simulink model "MDR_AA_TMD_Intercepteur"  (R2019b)
settings: Solver=ode4  StartTime=0.0  StopTime=Inf  FixedStep=0.01  RelTol=1e-3
values from neighbouring files (symbols this model uses):
  stdatm = [0 100 200 300 400 500 600 700 800 900 1000 1100 ... (4305 elements, 861x5)]    [stdatm.mat]
undefined symbols (not defined in the file or in its folder): Aero_Struct_CM, Aero_TMD, e0_0, e1_0, e2_0, e3_0, magnitude, Masse_Inertie_TMD, pow, Propu_TMD, Simu_TMD, Vm_0, xme_0
libraries: simulink x17
(part 1 of 4)
settings Model: Creator=julie  LastModifiedBy=julie

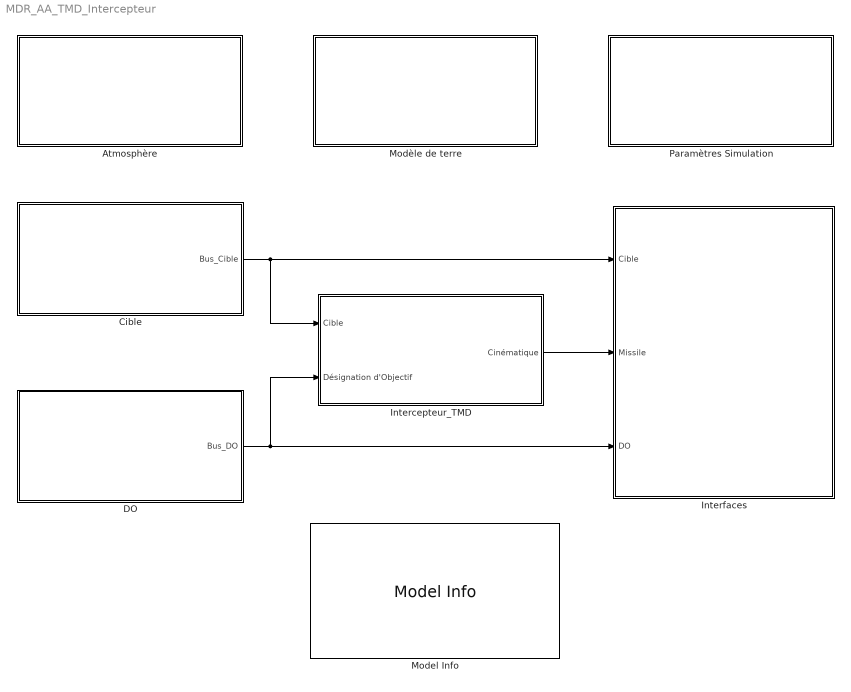
== system MDR_AA_TMD_Intercepteur ==
  Atmosphère : Subsystem
      mask Display: fprintf('Atmosphère')
  Cible : Subsystem  mask(Cible){}
      mask help: Evolution temporelle de la cible
      mask Display: fprintf('Cible')
  DO : Subsystem  mask(Cible){}
      mask help: Evolution temporelle de la DO
      mask Display: fprintf('Désignation d''Objectif')
  Intercepteur_TMD : Subsystem
      mask Display: fprintf('Missile')
  Interfaces : Subsystem
      mask Display: fprintf('Interfaces')
  Model Info : simulink/Model-Wide Utilities/Model Info  Frame=on  DisplayStringWithTags=|  HorizontalTextAlignment=Center  LeftAlignmentValue=0.5
      | Créé par Julien THADASACK
      | Modifié par 
      | %<ModifiedBy>
      | le 
      | %<ModifiedDate>
  Modèle de terre : Subsystem
      mask Display: fprintf('Modèle de terre')
  Paramètres Simulation : Subsystem
      mask Display: fprintf('Paramètres Simulation')
  wires:
  DO/1(Bus_DO) -> Intercepteur_TMD/2(Désignation d'Objectif), Interfaces/3(DO)
  Intercepteur_TMD/1(Cinématique) -> Interfaces/2(Missile)
  Cible/1(Bus_Cible) -> Intercepteur_TMD/1(Cible), Interfaces/1(Cible)

== system MDR_AA_TMD_Intercepteur/Atmosphère ==
  Atmosphère standard US76 : Subsystem  mask(Atmosphère standard US76){T_simu=-1}
      mask prompts: T_simu "Période de Simulation (s)"
      mask help: Recherche la pression, la température, la densité et la vitesse du son en fonction de l'altitude par rapport au niveau moyen de la mer.
      mask init:
      | load('stdatm');
      mask Help: eval('OpenHelp(''A3_NG.mdl'', ''\Help\html\A3_NG_Model_Atmosphere_US76.html'')');
  Bus Creator : BusCreator  Inputs=4
  Bus Selector : BusSelector  OutputSignals=Xi
  Selector : Selector  InputPortWidth=3  IndexOptions=Index vector (dialog)  Indices=[3]  OutputSizes=1
  Z positif vers le bas sinon : Gain  Gain=-1
  tag scope: Global_Atm=global
  wires:
  Atmosphère standard US76/3(Rho) -> Bus Creator/3  "Rho"
  Atmosphère standard US76/2(T) -> Bus Creator/2  "T"
  Atmosphère standard US76/4(Vson) -> Bus Creator/4  "Vson"
  Atmosphère standard US76/1(PS) -> Bus Creator/1  "PS"
  Bus Creator/1 -> [Global_Atm]
  [Global_Cine_Missile] -> Bus Selector/1
  Bus Selector/1 -> Selector/1  "<Xi>"
  Selector/1 -> Z positif vers le bas sinon/1
  Z positif vers le bas sinon/1 -> Atmosphère standard US76/1(Alt_MSL)

== system MDR_AA_TMD_Intercepteur/Cible ==
  Bus Creator : BusCreator  Inputs=2
  Cible Cinématique v1.1 : Subsystem  mask(Cible Cinématique v1.0){Pos_Init=[20000;0;-10000], Vit_Init=[-250;0;0], Az_Eva=[0 0], Tz_Eva=[0 1000], Ay_Eva=[0 0], Ty_Eva=[0 1000]}
      mask prompts: Pos_Init "Position initiale de la cible dans le repère inertiel NED [X;Y;Z] (en m)"; Vit_Init "Vitesse initiale de la cible dans le repère inertiel NED [Vx;Vy;Vz] (en m/s)"; Az_Eva "Table des accélérations commandée dans le plan de tangage (m/s²)"; Tz_Eva "Instants correspondant aux accélérations commandée dans le plan de tangage (en s)"; Ay_Eva "Table des accélérations commandée dans le plan de lacet (m/s²)"; Ty_Eva "Instants correspondant aux accélérations commandée dans le plan de lacet (en s)"
      mask help:
      | Modélisation de la trajectoire d'une cible cinématique (sans signature EM ou IR).
      |
      | Les mouvements de la cible sont définit à partir des accélérations commandées exprimées dans le repère cible en m/s².
      |
      | La vitesse de la cible reste constante au cours du vol et égale à la norme du vecteur vitesse initial.
      mask Help: eval('OpenHelp(''A3_NG.mdl'', ''Help\html\A3_NG_Model_Cible_v10.html'')');
  Bus_Cible : Outport  VectorParamsAs1DForOutWhenUnconnected=off
  tag scope: Global_Cible=global
  wires:
  Bus Creator/1 -> [Global_Cible], Bus_Cible/1  "Bus_Cible"
  Cible Cinématique v1.1/1(Vi) -> Bus Creator/1  "Vit_Cible"
  Cible Cinématique v1.1/2(Xi) -> Bus Creator/2  "Pos_Cible"

== system MDR_AA_TMD_Intercepteur/DO ==
  Ground : Ground
  Bus_DO : Outport  VectorParamsAs1DForOutWhenUnconnected=off
  wires:
  Ground/1 -> Bus_DO/1

== system MDR_AA_TMD_Intercepteur/Intercepteur_TMD ==
  Cible : Inport
  Désignation d'Objectif : Inport  Port=2
  Actionneurs : Subsystem  mask(Actionneurs){}
      mask help:
      | Fonctions transferts des actionneurs
      | alphaco -> alpha réalisé
      mask Display: fprintf('Actionneurs')
  Auto-Directeur : Subsystem  mask(Auto-Directeur){}
      mask Display: fprintf('Auto-Directeur')
  Bloc Cinématique : Subsystem  mask(Cinématique){}
      mask help: Calcul des accélérations, vitesses, positions et Euler à partir des forces et Euler
      mask Display: fprintf('Cinématique')
  Calculateur : Subsystem  mask(Calculateur){}
      mask help: Contient le logiciel embarqué dans la munition
      mask Display: fprintf('Calculateur')
  Forces-Moments : Subsystem  mask(Forces & Moments){}
      mask help: Calcul des forces aéro et de l'effet du vent
      mask Display: fprintf('Forces & Moments')
  Senseurs : Subsystem
      mask Display: fprintf('Senseurs')
  Structure : Subsystem  mask(Structure){}
      mask help: Calcul de l'évolution de la masse
      mask Display: fprintf('Structure')
  Cinématique : Outport  VectorParamsAs1DForOutWhenUnconnected=off
  wires:
  Calculateur/2(Actionneurs) -> Actionneurs/1(Bus_Pilote)
  Structure/1(Bus_Structure) -> Bloc Cinématique/1(Structure)
  Forces-Moments/1(Bus_ForcesMoments) -> Bloc Cinématique/2(Forces_Moments), Structure/1(Bus_Force_Moments)
  Actionneurs/1(Bus_Actionneurs_Miss) -> Forces-Moments/1(Bus_Actionneurs)
  Bloc Cinématique/1(Bus_Cine_Miss) -> Cinématique/1, Senseurs/1(Cinematique_Vrai), Auto-Directeur/2(Bus_Miss)
  Senseurs/1(Sorties_Capteurs) -> Calculateur/3(Senseurs)
  Auto-Directeur/1(Bus_AD_Miss) -> Calculateur/1(Auto-Directeur)
  Cible/1 -> Auto-Directeur/3(Bus_Cible)
  Désignation d'Objectif/1 -> Calculateur/2(Désignation d'Objectif)
  Calculateur/1(Superviseur) -> Auto-Directeur/1(Bus_Calculateur)

== system MDR_AA_TMD_Intercepteur/Interfaces ==
  note: VISUALISATION DE LA TRAJECTOIRE
  note: SORTIES DU MODELE
  Cible : Inport
  Missile : Inport  Port=2
  DO : Inport  Port=3
  Terminator : Terminator
  Terminator1 : Terminator
  Terminator2 : Terminator
  wires:
  Missile/1 -> Terminator/1
  Cible/1 -> Terminator1/1
  DO/1 -> Terminator2/1

== system MDR_AA_TMD_Intercepteur/Modèle de terre ==
  Bus Creator : BusCreator  Inputs=4
  Bus Selector : BusSelector  OutputSignals=Xi
  Modèle de terre WGS-84 : Subsystem  mask(WGS84){a=6378137, b=6356752.3142, gp=9.8321849378, ge=9.7803253359, GM=3986004.418e8, W=7.2921158553e-5, T_simu=-1}
      mask prompts: a "Earth equatorial radius (m):"; b "Earth polar radius (m):"; gp "Theoretical polar gravity (m/s²):"; ge "Theoretical equatorial gravity (m/s²):"; GM "Earth's Gravitationel Constant (Mass of Earth's atmosphere included) (m³/s²):"; W "Angular velocity of Earth (rad/s):"; T_simu "Periode de Simulation (s)"
      mask help: See Help.
      mask init:
      | % Compute 1st excentricity
      | e=sqrt((a^2-b^2)/a^2);
      | % Compute gravity formula constant
      | k=(b*gp)/(a*ge)-1;
      | m=W^2*a^2*b/GM;
      | % Compute ellipoidal flattening
      | f=(a-b)/a;
      mask Help: eval('OpenHelp(''A3_NG.mdl'', ''\Help\html\A3_NG_Model_Terre_WGS84.html'')');
  xyz_NED2LLA : Subsystem  mask(xyz_NED2LLA){LLA_Ref=[48.0333 -1.75 0], ellipsoid=[6378137 6356752.3142 0.08181919092891]}
      mask prompts: LLA_Ref "LLA de référence du repère TGL NED [deg deg m]"; ellipsoid "Ellispoïde"
      mask help: Calcul les coordonnées LLA (latitude, longitude, altitude) à partir des coordonnées xyz exprimées dans le repère NED (North, East, Down) dont l'origine du repère est définit par une position LLA de référence.
      mask Help: eval('OpenHelp(''A3_NG.mdl'', ''Help\html\A3_NG_Model_xyz_NED2LLA.html'')');
  tag scope: Global_Terre_Miss=global
  wires:
  Modèle de terre WGS-84/4(Gravity) -> Bus Creator/4  "g"
  Modèle de terre WGS-84/3(Re) -> Bus Creator/3  "Re"
  Modèle de terre WGS-84/2(Rnormal) -> Bus Creator/2  "Rn"
  Modèle de terre WGS-84/1(Rmeridian) -> Bus Creator/1  "Rm"
  Bus Creator/1 -> [Global_Terre_Miss]  "Bus_Terre"
  [Global_Cine_Missile] -> Bus Selector/1
  Bus Selector/1 -> xyz_NED2LLA/1(xyz_NED)  "<Xi>"
  xyz_NED2LLA/1(LLA) -> Modèle de terre WGS-84/1(LLA Position)

== system MDR_AA_TMD_Intercepteur/Paramètres Simulation ==
  Bus Selector : BusSelector  OutputSignals=Xi
  Bus Selector1 : BusSelector  OutputSignals=Pos_Cible
  Compare To Constant : simulink/Logic and Bit Operations/Compare To Constant  relop=<=  const=Simu_TMD.DDP_Min  OutDataTypeStr=boolean
  Impact Sol : simulink/Logic and Bit Operations/Compare To Zero  relop=>  OutDataTypeStr=boolean
  Logical Operator : Logic  Operator=OR  AllPortsSameDT=off  OutDataTypeStr=boolean
  Norme : Subsystem  mask(Norme){}
      mask help: Calcul la norme quadratique d'un vecteur.
      mask Help: eval('OpenHelp(''A3_NG.mdl'', ''Help\html\A3_NG_Model_Norme.html'')');
  Selector : Selector  InputPortWidth=3  IndexOptions=Index vector (dialog)  Indices=[3]  OutputSizes=1
  Stop Simulation : Stop
  Subtract : Sum  Inputs=+-
  wires:
  [Global_Cine_Missile] -> Bus Selector/1
  Bus Selector/1 -> Subtract/1, Selector/1  "<Xi>"
  Selector/1 -> Impact Sol/1
  Logical Operator/1 -> Stop Simulation/1
  Impact Sol/1 -> Logical Operator/1
  [Global_Cible] -> Bus Selector1/1
  Bus Selector1/1 -> Subtract/2  "<Pos_Cible>"
  Subtract/1 -> Norme/1(V)
  Norme/1(||V||) -> Compare To Constant/1
  Compare To Constant/1 -> Logical Operator/2

== system MDR_AA_TMD_Intercepteur/Atmosphère/Atmosphère standard US76 ==
  note: 1976 Standard Atmosphere Look-up Tables
  Alt_MSL : Inport  PortDimensions=1
  Density LUT : Lookup  InputValues=stdatm(:,1)  Table=stdatm(:,4)  SaturateOnIntegerOverflow=on
  Pressure LUT : Lookup  InputValues=stdatm(:,1)  Table=stdatm(:,3)  SaturateOnIntegerOverflow=on
  Saturation : Saturate  UpperLimit=86000  LowerLimit=0
  Speed of sound LUT : Lookup  InputValues=stdatm(:,1)  Table=stdatm(:,5)  SaturateOnIntegerOverflow=on
  Temperature LUT : Lookup  InputValues=stdatm(:,1)  Table=stdatm(:,2)  SaturateOnIntegerOverflow=on
  PS : Outport  VectorParamsAs1DForOutWhenUnconnected=off
  T : Outport  Port=2  VectorParamsAs1DForOutWhenUnconnected=off
  Rho : Outport  Port=3  VectorParamsAs1DForOutWhenUnconnected=off
  Vson : Outport  Port=4  VectorParamsAs1DForOutWhenUnconnected=off
  wires:
  Speed of sound LUT/1 -> Vson/1
  Pressure LUT/1 -> PS/1
  Temperature LUT/1 -> T/1
  Saturation/1 -> Density LUT/1, Speed of sound LUT/1, Pressure LUT/1, Temperature LUT/1
  Density LUT/1 -> Rho/1
  Alt_MSL/1 -> Saturation/1

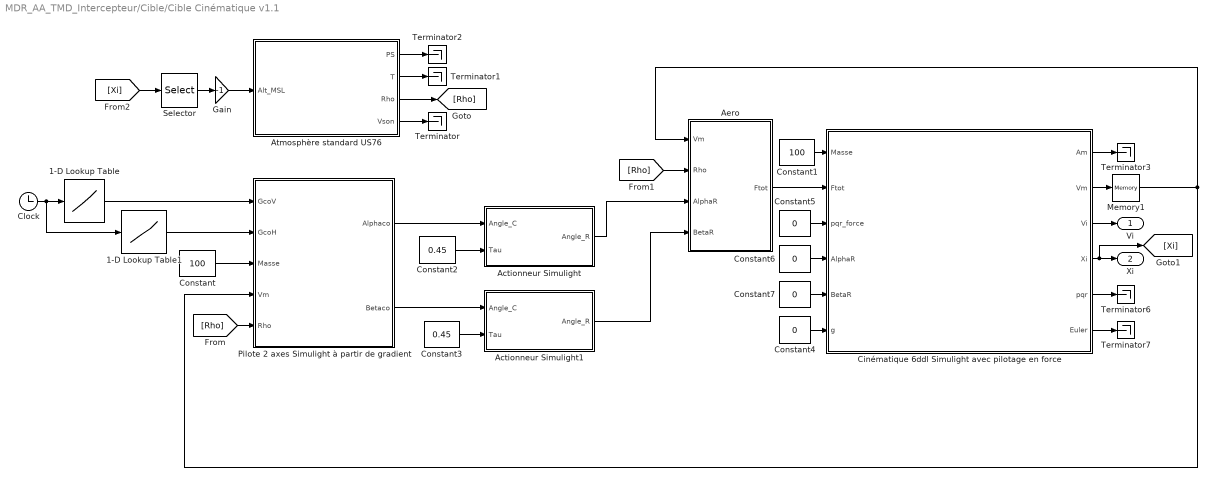
== system MDR_AA_TMD_Intercepteur/Cible/Cible Cinématique v1.1 ==
  1-D Lookup Table : Lookup_n-D  NumberOfTableDimensions=1  BreakpointsForDimension1=Tz_Eva  Table=Az_Eva  RndMeth=Simplest  InputSameDT=on
  1-D Lookup Table1 : Lookup_n-D  NumberOfTableDimensions=1  BreakpointsForDimension1=Ty_Eva  Table=Ay_Eva  RndMeth=Simplest  InputSameDT=on
  Actionneur Simulight : Subsystem  mask(Actionneur de type Simulight){ShowInLibBrowser=0}
      mask prompts: ShowInLibBrowser "Simulink:masks:ActSimu"
      mask help:
      | Modèle de pseudo actionneur appliquant un temps de réponse à la commande envoyée par le pilote.
      |
      | Le modèle d'actionneur de Simulight est assimilable à une fonction du premier ordre de temps de réponse Tau.
      |
      | Tau représente le temps de réponse global du missile.
      mask Help: eval('OpenHelp(''A3_NG.mdl'', ''Help\html\A3_NG_Model_Actionneur_Simulight.html'')');
  Actionneur Simulight1 : Subsystem  mask(Actionneur de type Simulight){ShowInLibBrowser=0}
      mask prompts: ShowInLibBrowser "Simulink:masks:ActSimu"
      mask help:
      | Modèle de pseudo actionneur appliquant un temps de réponse à la commande envoyée par le pilote.
      |
      | Le modèle d'actionneur de Simulight est assimilable à une fonction du premier ordre de temps de réponse Tau.
      |
      | Tau représente le temps de réponse global du missile.
      mask Help: eval('OpenHelp(''A3_NG.mdl'', ''Help\html\A3_NG_Model_Actionneur_Simulight.html'')');
  Aero : Subsystem  mask{Lref=0.200, Cza=0.5, Cyb=0.5}
      mask prompts: Lref "Longueur de référence (en m)"; Cza "Gradient de protance Cza"; Cyb "Gradient de portance Cyb"
  Atmosphère standard US76 : Subsystem  mask(Atmosphère standard US76){T_simu=-1}
      mask prompts: T_simu "Période de Simulation (s)"
      mask help: Recherche la pression, la température, la densité et la vitesse du son en fonction de l'altitude par rapport au niveau moyen de la mer.
      mask init:
      | load('stdatm');
      mask Help: eval('OpenHelp(''A3_NG.mdl'', ''\Help\html\A3_NG_Model_Atmosphere_US76.html'')');
  Cinématique 6ddl Simulight avec pilotage en force : Subsystem  mask(Bloc Cinématique 6DDL Simulight avec pilotage en force){Vb0=Vit_Init, pqr0=[0;0;0], Xe0=Pos_Init, Euler_Init=[0;0;0], Longueur_Missile=0}
      mask prompts: Vb0 "Vitesse initiale (repère missile)"; pqr0 "Vitesse de rotation initiale"; Xe0 "Position initiale (repère inertiel)"; Euler_Init "Angles d'Euler initiaux"; Longueur_Missile "Longueur Missile (en mm)"
      mask help:
      | Bloc cinématique 6DDL
      |
      | ENTREES
      | Masse: Masse du missile (1x1)
      | Ftot: Somme des forces extèrieures au missile (3x1)
      | pqr_force: Vitesse de rotation induite par du pilotage en force (3x1)
      | AlphaR: Incidence réalisée au sens de simulight (1x1)
      | BetaR: Dérapage réalisé au sens de simulight (1x1)
      | g: Gravité exprimée à la position du missile (1x1)
      |
      | SORTIES
      | Am: Accélération du missile exprimés dans le repère missile (3x1)
      | Vm: Vitesse du missile exprimée dans le repère missile (3x1)
      | Vi: Vitesse du missile exprimée dans le repère inertiel (3x1)
      | Xi: Position du missile exprimée dans le repère inertiel (3x1)
      | pqr: Vitesse de rotation angulaire du missile (3x1)
      | Euler: Angles d'Euler du missile (3x1)
      mask Help: eval('OpenHelp(''A3_NG.mdl'', ''Help\html\A3_NG_Model_Cinematique_6ulight_PIF.html'')');
  Clock : Clock
  Constant : Constant  Value=100
  Constant1 : Constant  Value=100
  Constant2 : Constant  Value=0.45
  Constant3 : Constant  Value=0.45
  Constant{4..7} (4 alike) : Constant  Value=0
  Gain : Gain  Gain=-1
  Memory1 : Memory
  Pilote 2 axes Simulight à partir de gradient : Subsystem  mask(Pilote 2 axes Simulight){Lref=0.200, Cza=0.5, Cyb=0.5}
      mask prompts: Lref "Longeur de référence (m)"; Cza "Gradient de portance Cza"; Cyb "Gradient de portance Cyb"
      mask help: Calcul de l'incidence et du dérapage commandés permettant d'atteindre la consigne envoyée par le guidage.
      mask Help: eval('OpenHelp(''A3_NG.mdl'', ''Help\html\A3_NG_Model_Pilote_2axes_Simulight.html'')');
  Selector : Selector  InputPortWidth=3  IndexOptions=Index vector (dialog)  Indices=[3]  OutputSizes=1
  Terminator{,1..3,6..7} (6 alike) : Terminator
  Vi : Outport  VectorParamsAs1DForOutWhenUnconnected=off
  Xi : Outport  Port=2  VectorParamsAs1DForOutWhenUnconnected=off
  wires:
  Cinématique 6ddl Simulight avec pilotage en force/4(Xi) -> [Xi], Xi/1
  Constant7/1 -> Cinématique 6ddl Simulight avec pilotage en force/5(BetaR)
  Constant6/1 -> Cinématique 6ddl Simulight avec pilotage en force/4(AlphaR)
  1-D Lookup Table1/1 -> Pilote 2 axes Simulight à partir de gradient/2(GcoH)
  1-D Lookup Table/1 -> Pilote 2 axes Simulight à partir de gradient/1(GcoV)
  Clock/1 -> 1-D Lookup Table1/1, 1-D Lookup Table/1
  Aero/1(Ftot) -> Cinématique 6ddl Simulight avec pilotage en force/2(Ftot)
  Memory1/1 -> Pilote 2 axes Simulight à partir de gradient/4(Vm), Aero/1(Vm)
  Gain/1 -> Atmosphère standard US76/1(Alt_MSL)
  Selector/1 -> Gain/1
  [Xi] -> Selector/1
  Constant5/1 -> Cinématique 6ddl Simulight avec pilotage en force/3(pqr_force)
  Cinématique 6ddl Simulight avec pilotage en force/6(Euler) -> Terminator7/1
  Cinématique 6ddl Simulight avec pilotage en force/5(pqr) -> Terminator6/1
  Cinématique 6ddl Simulight avec pilotage en force/3(Vi) -> Vi/1
  Cinématique 6ddl Simulight avec pilotage en force/1(Am) -> Terminator3/1
  [Rho] -> Aero/2(Rho)
  [Rho] -> Pilote 2 axes Simulight à partir de gradient/5(Rho)
  Atmosphère standard US76/1(PS) -> Terminator2/1
  Atmosphère standard US76/2(T) -> Terminator1/1
  Atmosphère standard US76/4(Vson) -> Terminator/1
  Atmosphère standard US76/3(Rho) -> [Rho]
  Constant4/1 -> Cinématique 6ddl Simulight avec pilotage en force/6(g)
  Actionneur Simulight1/1(Angle_R) -> Aero/4(BetaR)
  Actionneur Simulight/1(Angle_R) -> Aero/3(AlphaR)
  Constant3/1 -> Actionneur Simulight1/2(Tau)
  Constant2/1 -> Actionneur Simulight/2(Tau)
  Cinématique 6ddl Simulight avec pilotage en force/2(Vm) -> Memory1/1
  Constant1/1 -> Cinématique 6ddl Simulight avec pilotage en force/1(Masse)
  Constant/1 -> Pilote 2 axes Simulight à partir de gradient/3(Masse)
  Pilote 2 axes Simulight à partir de gradient/2(Betaco) -> Actionneur Simulight1/1(Angle_C)
  Pilote 2 axes Simulight à partir de gradient/1(Alphaco) -> Actionneur Simulight/1(Angle_C)

== system MDR_AA_TMD_Intercepteur/Intercepteur_TMD/Actionneurs ==
  note: Modèle d'actionneur à ajouter
  Bus_Pilote : Inport
  Bus Creator : BusCreator  Inputs=2
  Bus Selector : BusSelector  OutputSignals=AlphaC,BetaC
  Bus_Actionneurs_Miss : Outport  VectorParamsAs1DForOutWhenUnconnected=off
  tag scope: Global_Actionneurs=global
  wires:
  Bus_Pilote/1 -> Bus Selector/1
  Bus Selector/2 -> Bus Creator/2  "<BetaC>"
  Bus Selector/1 -> Bus Creator/1  "<AlphaC>"
  Bus Creator/1 -> [Global_Actionneurs], Bus_Actionneurs_Miss/1  "Bus_Actionneurs"

== system MDR_AA_TMD_Intercepteur/Intercepteur_TMD/Auto-Directeur ==
  Bus_Calculateur : Inport
  Bus_Miss : Inport  Port=2
  Bus_Cible : Inport  Port=3
  Autodirecteur Parfait v1.0 : Subsystem  mask(Autodirecteur Parfait v1.0){}
      mask help:
      | Modèle d'autodirecteur parfait donnant:
      | - Les vitesses de défilements selon deux plans
      | - Les écartométries selon deux plans
      | - Le dépointage total de la ligne de visée par rapport à l'axe missile
      mask Help: eval('OpenHelp(''A3_NG.mdl'', ''Help\html\A3_NG_Model_AD_Parfait_v10.html'')');
  Bus Creator : BusCreator  Inputs=5
  Bus Selector : BusSelector  OutputSignals=Pos_Cible,Vit_Cible
  Bus Selector1 : BusSelector  OutputSignals=Senseur.Xi,Senseur.Vi
  Bus Selector2 : BusSelector  OutputSignals=Euler
  Bus_AD_Miss : Outport  VectorParamsAs1DForOutWhenUnconnected=off
  wires:
  Bus_Calculateur/1 -> Bus Selector1/1
  Bus_Cible/1 -> Bus Selector/1
  Autodirecteur Parfait v1.0/4(Theta_ad) -> Bus Creator/4  "Theta_ad"
  Autodirecteur Parfait v1.0/3(Psi_ad) -> Bus Creator/3  "Psi_ad"
  Autodirecteur Parfait v1.0/5(Lambda_ad) -> Bus Creator/5  "Lambda_ad"
  Autodirecteur Parfait v1.0/2(Lambda_pt_z) -> Bus Creator/2  "Lambda_pt_z"
  Autodirecteur Parfait v1.0/1(Lambda_pt_y) -> Bus Creator/1  "Lambda_pt_y"
  Bus Creator/1 -> Bus_AD_Miss/1  "Bus_AD"
  Bus Selector/2 -> Autodirecteur Parfait v1.0/2(Vit_Cible)  "<Vit_Cible>"
  Bus Selector/1 -> Autodirecteur Parfait v1.0/1(Pos_Cible)  "<Pos_Cible>"
  Bus Selector1/1 -> Autodirecteur Parfait v1.0/3(Pos_Miss)  "<Xi>"
  Bus Selector1/2 -> Autodirecteur Parfait v1.0/4(Vit_Miss)  "<Vi>"
  Bus_Miss/1 -> Bus Selector2/1
  Bus Selector2/1 -> Autodirecteur Parfait v1.0/5(Euler)  "<Euler>"

== system MDR_AA_TMD_Intercepteur/Intercepteur_TMD/Bloc Cinématique ==
  Structure : Inport
  Forces_Moments : Inport  Port=2
  Add : Sum
  Bus Creator : BusCreator  Inputs=6
  Bus Selector : BusSelector  OutputSignals=Faero,Fpropu
  Bus Selector1 : BusSelector  OutputSignals=Masse
  Bus Selector2 : BusSelector  OutputSignals=AlphaC,BetaC
  Bus Selector3 : BusSelector  OutputSignals=g
  Cinématique 6ddl Simulight avec pilotage en force : Subsystem  mask(Bloc Cinématique 6DDL Simulight avec pilotage en force){Vb0=[284.4288             0             0], pqr0=[0;0;0], Xe0=[-10000           0           0], Euler_Init=[0  10  0], Longueur_Missile=4000}
      mask prompts: Vb0 "Vitesse initiale (repère missile)"; pqr0 "Vitesse de rotation initiale"; Xe0 "Position initiale (repère inertiel)"; Euler_Init "Angles d'Euler initiaux"; Longueur_Missile "Longueur Missile (en mm)"
      mask help:
      | Bloc cinématique 6DDL
      |
      | ENTREES
      | Masse: Masse du missile (1x1)
      | Ftot: Somme des forces extèrieures au missile (3x1)
      | pqr_force: Vitesse de rotation induite par du pilotage en force (3x1)
      | AlphaR: Incidence réalisée au sens de simulight (1x1)
      | BetaR: Dérapage réalisé au sens de simulight (1x1)
      | g: Gravité exprimée à la position du missile (1x1)
      |
      | SORTIES
      | Am: Accélération du missile exprimés dans le repère missile (3x1)
      | Vm: Vitesse du missile exprimée dans le repère missile (3x1)
      | Vi: Vitesse du missile exprimée dans le repère inertiel (3x1)
      | Xi: Position du missile exprimée dans le repère inertiel (3x1)
      | pqr: Vitesse de rotation angulaire du missile (3x1)
      | Euler: Angles d'Euler du missile (3x1)
      mask Help: eval('OpenHelp(''A3_NG.mdl'', ''Help\html\A3_NG_Model_Cinematique_6ulight_PIF.html'')');
  Ground : Ground
  Bus_Cine_Miss : Outport  VectorParamsAs1DForOutWhenUnconnected=off
  tag scope: Global_Cine_Missile=global
  wires:
  Bus Creator/1 -> [Global_Cine_Missile], Bus_Cine_Miss/1  "Bus_Cine"
  Cinématique 6ddl Simulight avec pilotage en force/4(Xi) -> Bus Creator/4  "Xi"
  Cinématique 6ddl Simulight avec pilotage en force/3(Vi) -> Bus Creator/3  "Vi"
  Cinématique 6ddl Simulight avec pilotage en force/5(pqr) -> Bus Creator/5  "pqr"
  Cinématique 6ddl Simulight avec pilotage en force/2(Vm) -> Bus Creator/2  "Vm"
  Cinématique 6ddl Simulight avec pilotage en force/6(Euler) -> Bus Creator/6  "Euler"
  Cinématique 6ddl Simulight avec pilotage en force/1(Am) -> Bus Creator/1  "Am"
  Forces_Moments/1 -> Bus Selector/1
  Bus Selector/1 -> Add/1  "<Faero>"
  Bus Selector/2 -> Add/2  "<Fpropu>"
  Add/1 -> Cinématique 6ddl Simulight avec pilotage en force/2(Ftot)
  Ground/1 -> Cinématique 6ddl Simulight avec pilotage en force/3(pqr_force)
  Structure/1 -> Bus Selector1/1
  Bus Selector1/1 -> Cinématique 6ddl Simulight avec pilotage en force/1(Masse)  "<Masse>"
  [Global_Actionneurs] -> Bus Selector2/1
  Bus Selector2/1 -> Cinématique 6ddl Simulight avec pilotage en force/4(AlphaR)  "<AlphaC>"
  Bus Selector2/2 -> Cinématique 6ddl Simulight avec pilotage en force/5(BetaR)  "<BetaC>"
  [Global_Terre_Miss] -> Bus Selector3/1
  Bus Selector3/1 -> Cinématique 6ddl Simulight avec pilotage en force/6(g)  "<g>"

== system MDR_AA_TMD_Intercepteur/Intercepteur_TMD/Calculateur ==
  Auto-Directeur : Inport
  Désignation d'Objectif : Inport  Port=2
  Senseurs : Inport  Port=3
  Bloc Superviseur : Subsystem
      mask Display: fprintf('Superviseur')
  Guidage : Subsystem
      mask Display: fprintf('Guidage')
  Pilotage : Subsystem  mask(Pilotage){}
      mask help: Calcul des alfaco et betaco à partir des accélérations commandées
      mask Display: fprintf('Pilotage')
  Préparation de mission : Subsystem
      mask Display: fprintf('Préparation de mission')
  Superviseur : Outport  VectorParamsAs1DForOutWhenUnconnected=off
  Actionneurs : Outport  Port=2  VectorParamsAs1DForOutWhenUnconnected=off
  wires:
  Préparation de mission/1(Bus_PM) -> Bloc Superviseur/1(Bus_PM)
  Auto-Directeur/1 -> Bloc Superviseur/2(Bus_AD)
  Désignation d'Objectif/1 -> Bloc Superviseur/3(Bus_DO)
  Bloc Superviseur/1(Bus_Superviseur) -> Guidage/1(Bus_Superviseur), Superviseur/1
  Guidage/1(Bus_Guidage) -> Pilotage/1(Bus_Guidage)
  Pilotage/1(Bus_Pilote) -> Actionneurs/1
  Senseurs/1 -> Bloc Superviseur/4(Bus_Senseurs)

== system MDR_AA_TMD_Intercepteur/Intercepteur_TMD/Forces-Moments ==
  Bus_Actionneurs : Inport
  Aerodynamique 3D (CA/CY/CN) v1.0 : Subsystem  mask(Aérodynamique 3D (CA/CY/CN) v1.0){vMach=Aero_TMD.vMach, vAlt=Aero_TMD.vAlt, vAlpha=Aero_TMD.vAlpha, vBeta=Aero_TMD.vBeta, Lref=Aero_TMD.Lref, CA_np=Aero_TMD.CA_np, CA_p=Aero_TMD.CA_p, CY=Aero_TMD.CY, CN=Aero_TMD.CN}
      mask prompts: vMach "Valeurs de Mach de l'étude"; vAlt "Valeurs d'altitude de l'étude (m)"; vAlpha "Valeurs d'incidence de l'étude (°)"; vBeta "Valeurs de dérapage de l'étude (°)"; Lref "Longueur de référence (m)"; CA_np "Matrice des coefficients de trainée non propulsée (CA_np)"; CA_p "Matrice des coefficients de trainée propulsée (CA_p)"; CY "Matrice des coefficients de portance (CY)"; CN "Matrice des coefficients de portance (CN)"
      mask help: Calcul des efforts aérodynamique à partir des coefficients CA/CY/CN.
      mask Help: eval('OpenHelp(''A3_NG.mdl'', ''Help\html\A3_NG_Model_Aero_3D_v10.html'')');
  Bus Creator : BusCreator  Inputs=3
  Bus Selector : BusSelector  OutputSignals=Xi,Vm
  Bus Selector1 : BusSelector  OutputSignals=Rho,Vson
  Bus Selector2 : BusSelector  OutputSignals=AlphaC,BetaC
  Bus Selector3 : BusSelector  OutputSignals=PS
  Gain : Gain  Gain=-1
  Propulsion de l'exemple TMD : Subsystem
  Selector : Selector  InputPortWidth=3  IndexOptions=Index vector (dialog)  Indices=[3]  OutputSizes=1
  Sum of Elements : Sum  Inputs=+
  Bus_ForcesMoments : Outport  VectorParamsAs1DForOutWhenUnconnected=off
  wires:
  Bus Creator/1 -> Bus_ForcesMoments/1
  Aerodynamique 3D (CA/CY/CN) v1.0/1(Faero) -> Bus Creator/1  "Faero"
  [Global_Cine_Missile] -> Bus Selector/1
  Bus Selector/1 -> Selector/1  "<Xi>"
  Bus Selector/2 -> Aerodynamique 3D (CA/CY/CN) v1.0/2(Vm)  "<Vm>"
  Selector/1 -> Gain/1
  Gain/1 -> Aerodynamique 3D (CA/CY/CN) v1.0/1(Altitude)
  [Global_Atm] -> Bus Selector3/1, Bus Selector1/1
  Bus Selector1/1 -> Aerodynamique 3D (CA/CY/CN) v1.0/3(Rho)  "<Rho>"
  Bus Selector1/2 -> Aerodynamique 3D (CA/CY/CN) v1.0/4(Vson)  "<Vson>"
  Bus_Actionneurs/1 -> Bus Selector2/1
  Bus Selector2/1 -> Aerodynamique 3D (CA/CY/CN) v1.0/5(AlphaR)  "<AlphaC>"
  Bus Selector2/2 -> Aerodynamique 3D (CA/CY/CN) v1.0/6(BetaR)  "<BetaC>"
  Bus Selector3/1 -> Propulsion de l'exemple TMD/1(<PS>)  "<PS>"
  Propulsion de l'exemple TMD/1(Fpropu) -> Bus Creator/2, Sum of Elements/1  "Fpropu"
  Propulsion de l'exemple TMD/2(debit_carburant) -> Bus Creator/3  "debit_carburant"
  Sum of Elements/1 -> Aerodynamique 3D (CA/CY/CN) v1.0/7(Ok_propu)

== system MDR_AA_TMD_Intercepteur/Intercepteur_TMD/Senseurs ==
  Cinematique_Vrai : Inport
  Bus Creator : BusCreator  Inputs=6
  Bus Selector : BusSelector  OutputSignals=Am,Vm,Vi,Xi,pqr,Euler
  Sorties_Capteurs : Outport  VectorParamsAs1DForOutWhenUnconnected=off
  wires:
  Cinematique_Vrai/1 -> Bus Selector/1
  Bus Creator/1 -> Sorties_Capteurs/1  "Bus_Capteurs"
  Bus Selector/4 -> Bus Creator/4  "<Xi>"
  Bus Selector/3 -> Bus Creator/3  "<Vi>"
  Bus Selector/5 -> Bus Creator/5  "<pqr>"
  Bus Selector/2 -> Bus Creator/2  "<Vm>"
  Bus Selector/6 -> Bus Creator/6  "<Euler>"
  Bus Selector/1 -> Bus Creator/1  "<Am>"

== system MDR_AA_TMD_Intercepteur/Intercepteur_TMD/Structure ==
  Bus_Force_Moments : Inport
  Bus Creator : BusCreator  Inputs=1
  Bus Selector : BusSelector  OutputSignals=debit_carburant
  Integrator : Integrator
  Masse Initiale : Constant  Value=Masse_Inertie_TMD.Masse_Init
  Subtract : Sum  Inputs=+-
  Bus_Structure : Outport  VectorParamsAs1DForOutWhenUnconnected=off
  tag scope: Global_Structure=global
  wires:
  Bus_Force_Moments/1 -> Bus Selector/1
  Bus Selector/1 -> Integrator/1  "<debit_carburant>"
  Masse Initiale/1 -> Subtract/1
  Integrator/1 -> Subtract/2
  Subtract/1 -> Bus Creator/1  "Masse"
  Bus Creator/1 -> [Global_Structure], Bus_Structure/1  "Bus_Structure"

== system MDR_AA_TMD_Intercepteur/Modèle de terre/Modèle de terre WGS-84 ==
  note: Latitude
  note: Longitude
  LLA Position : Inport
  Computation of Earth curvature radius (WGS-84) : Subsystem
  Computation of the local gravity : Subsystem
  Demux : Demux  Outputs=3
  Terminator : Terminator
  Rmeridian : Outport  VectorParamsAs1DForOutWhenUnconnected=off
  Rnormal : Outport  Port=2  VectorParamsAs1DForOutWhenUnconnected=off
  Re : Outport  Port=3  VectorParamsAs1DForOutWhenUnconnected=off
  Gravity : Outport  Port=4  VectorParamsAs1DForOutWhenUnconnected=off
  wires:
  Computation of Earth curvature radius (WGS-84)/2(Rnormal) -> Rnormal/1
  Computation of Earth curvature radius (WGS-84)/1(Rmeridian) -> Rmeridian/1
  Demux/1 -> Computation of Earth curvature radius (WGS-84)/1(Latitude), Computation of the local gravity/1(Latitude)
  Computation of Earth curvature radius (WGS-84)/3(Re) -> Re/1
  Demux/2 -> Terminator/1
  Demux/3 -> Computation of the local gravity/2(Altitude)  "Altitude"
  LLA Position/1 -> Demux/1
  Computation of the local gravity/1(Gravity) -> Gravity/1

== system MDR_AA_TMD_Intercepteur/Modèle de terre/xyz_NED2LLA ==
  xyz_NED : Inport
  ECEF2LLA : Subsystem  mask(ECEF2LLA){a=6378137, b=6356752.3142, e=0.08181919092891}
      mask prompts: a "1/2 grand axe equatorial de l'ellipsoïde"; b "1/2 grand axe polaire de l'ellipsoïde"; e "Excentricité de l'ellipsoïde"
      mask help: Transforme les coordonnées dans le repère ECEF (Earth-Centered Earth Fixed) [m,m,m] en coordonnées géographiques LLA [rad,rad,m] par rapport à l'ellipsoïde de référence)
      mask Help: eval('OpenHelp(''A3_NG.mdl'', ''Help\html\A3_NG_Model_ECEF2LLA.html'')');
  END2ENU : Gain  Gain=[1;1;-1]
  NED2END : Selector  InputPortWidth=3  IndexOptions=Index vector (dialog)  Indices=[2 1 3]  OutputSizes=1
  xyz_ENU2ECEF : Subsystem  mask(xyz_ENU2ECEF){Phi0=LLA_Ref(1), Lambda0=LLA_Ref(2), h0=LLA_Ref(3), a=6378137, b=6356752.3142, e=0.08181919092891}
      mask prompts: Phi0 "Latitude de référence du repère TGL NED (deg)"; Lambda0 "Longitude de référence du repère TGL NED (deg)"; h0 "Altitude de référence du repère TGL NED (m)"; a "1/2 grand axe equatorial de l'ellipsoïde"; b "1/2 grand axe polaire de l'ellipsoïde"; e "Excentricité de l'ellipsoïde"
      mask help: Transforme les coordonnées dans le repère ENU local (East North Up) xyz= [m,m,m] défini par le plan tangent à l'ellipsoïde au point origine lla0 [rad,rad,m] et le vecteur normal défini positivement suivant les altitudes dans le repère ECEF (Earth Centered Earth Fixed).
      mask init:
      | Phi0 = Phi0*pi/180;
      | Lambda0 = Lambda0*pi/180;
      mask Help: eval('OpenHelp(''A3_NG.mdl'', ''Help\html\A3_NG_Model_xyz_ENU2ECEF.html'')');
  LLA : Outport  VectorParamsAs1DForOutWhenUnconnected=off
  wires:
  ECEF2LLA/1(LLA) -> LLA/1
  xyz_NED/1 -> NED2END/1
  xyz_ENU2ECEF/1(ECEF) -> ECEF2LLA/1(ECEF)
  NED2END/1 -> END2ENU/1
  END2ENU/1 -> xyz_ENU2ECEF/1(xyz_ENU)

== system MDR_AA_TMD_Intercepteur/Paramètres Simulation/Norme ==
  V : Inport
  Dot Product : DotProduct  InputSameDT=on  OutDataTypeStr=Inherit: Inherit via internal rule
  Sqrt : Math  Operator=sqrt  SaturateOnIntegerOverflow=on
  ||V|| : Outport  VectorParamsAs1DForOutWhenUnconnected=off
  wires:
  Sqrt/1 -> ||V||/1
  V/1 -> Dot Product/2, Dot Product/1
  Dot Product/1 -> Sqrt/1

== system MDR_AA_TMD_Intercepteur/Cible/Cible Cinématique v1.1/Actionneur Simulight ==
  Angle_C : Inport
  Tau : Inport  Port=2
  Memory : Memory  InheritSampleTime=on
  Retard Angle : Subsystem
  Angle_R : Outport  VectorParamsAs1DForOutWhenUnconnected=off
  wires:
  Retard Angle/1(Angle_R) -> Angle_R/1, Memory/1
  Memory/1 -> Retard Angle/1(Angle_t_1)
  Angle_C/1 -> Retard Angle/2(Angle_C)
  Tau/1 -> Retard Angle/3(Tau)

== system MDR_AA_TMD_Intercepteur/Cible/Cible Cinématique v1.1/Actionneur Simulight1 ==
  Angle_C : Inport
  Tau : Inport  Port=2
  Memory : Memory  InheritSampleTime=on
  Retard Angle : Subsystem
  Angle_R : Outport  VectorParamsAs1DForOutWhenUnconnected=off
  wires:
  Retard Angle/1(Angle_R) -> Angle_R/1, Memory/1
  Memory/1 -> Retard Angle/1(Angle_t_1)
  Angle_C/1 -> Retard Angle/2(Angle_C)
  Tau/1 -> Retard Angle/3(Tau)

== system MDR_AA_TMD_Intercepteur/Cible/Cible Cinématique v1.1/Aero ==
  Vm : Inport
  Rho : Inport  Port=2
  AlphaR : Inport  Port=3
  BetaR : Inport  Port=4
  Constant : Constant  Value=0
  Cyb : Gain  Gain=Cyb
  Cza : Gain  Gain=Cza
  Norme : Subsystem  mask(Norme){}
      mask help: Calcul la norme quadratique d'un vecteur.
      mask Help: eval('OpenHelp(''A3_NG.mdl'', ''Help\html\A3_NG_Model_Norme.html'')');
  Product : Product  RndMeth=Zero
  Product1 : Product  RndMeth=Zero
  Vector Concatenate : Concatenate  NumInputs=3
  q\ : Subsystem
  Ftot : Outport  VectorParamsAs1DForOutWhenUnconnected=off
  wires:
  Cza/1 -> Product1/2
  Cyb/1 -> Product/1
  Constant/1 -> Vector Concatenate/1
  Product/1 -> Vector Concatenate/2
  Product1/1 -> Vector Concatenate/3
  Vector Concatenate/1 -> Ftot/1
  q\/1(rsv2) -> Product1/1, Product/2
  AlphaR/1 -> Cza/1
  BetaR/1 -> Cyb/1
  Vm/1 -> Norme/1(V)
  Rho/1 -> q\/2(Rho)
  Norme/1(||V||) -> q\/1(||V||)

== system MDR_AA_TMD_Intercepteur/Cible/Cible Cinématique v1.1/Atmosphère standard US76 ==
  note: 1976 Standard Atmosphere Look-up Tables
  Alt_MSL : Inport  PortDimensions=1
  Density LUT : Lookup  InputValues=stdatm(:,1)  Table=stdatm(:,4)  SaturateOnIntegerOverflow=on
  Pressure LUT : Lookup  InputValues=stdatm(:,1)  Table=stdatm(:,3)  SaturateOnIntegerOverflow=on
  Saturation : Saturate  UpperLimit=86000  LowerLimit=0
  Speed of sound LUT : Lookup  InputValues=stdatm(:,1)  Table=stdatm(:,5)  SaturateOnIntegerOverflow=on
  Temperature LUT : Lookup  InputValues=stdatm(:,1)  Table=stdatm(:,2)  SaturateOnIntegerOverflow=on
  PS : Outport  VectorParamsAs1DForOutWhenUnconnected=off
  T : Outport  Port=2  VectorParamsAs1DForOutWhenUnconnected=off
  Rho : Outport  Port=3  VectorParamsAs1DForOutWhenUnconnected=off
  Vson : Outport  Port=4  VectorParamsAs1DForOutWhenUnconnected=off
  wires:
  Speed of sound LUT/1 -> Vson/1
  Pressure LUT/1 -> PS/1
  Temperature LUT/1 -> T/1
  Saturation/1 -> Density LUT/1, Speed of sound LUT/1, Pressure LUT/1, Temperature LUT/1
  Density LUT/1 -> Rho/1
  Alt_MSL/1 -> Saturation/1

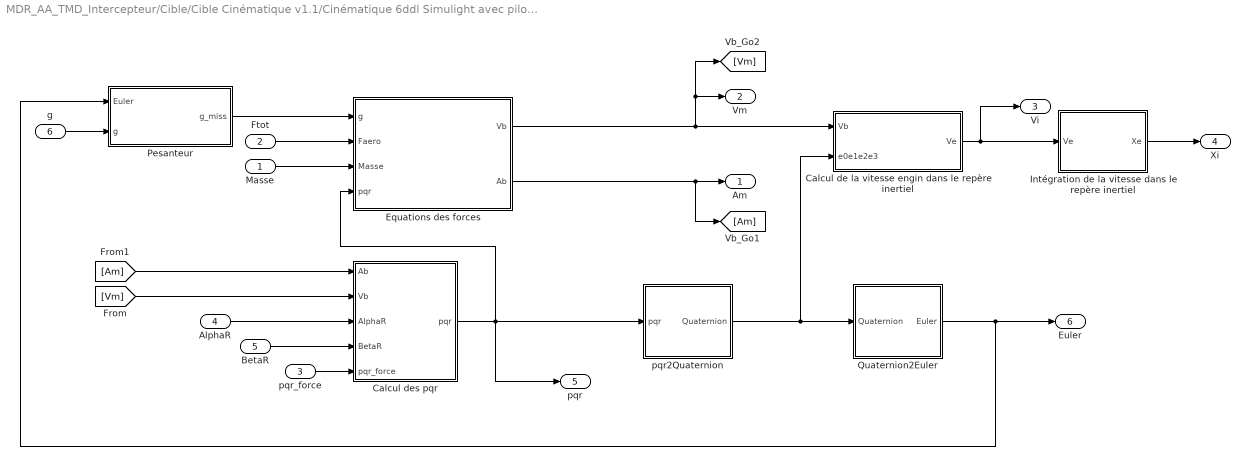
== system MDR_AA_TMD_Intercepteur/Cible/Cible Cinématique v1.1/Cinématique 6ddl Simulight avec pilotage en force ==
  Masse : Inport
  Ftot : Inport  Port=2
  pqr_force : Inport  Port=3
  AlphaR : Inport  Port=4
  BetaR : Inport  Port=5
  g : Inport  Port=6
  Calcul de la vitesse engin dans le repère inertiel : Subsystem
  Calcul des pqr : Subsystem
  Equations des forces : Subsystem
  Intégration de la vitesse dans le repère inertiel : Subsystem
  Pesanteur : Subsystem
  Quaternion2Euler : Subsystem  mask(Quaternion2Euler){}
      mask help:
      | Calcul des angles d'Euler (phi,theta,psi) à partir du quaternion q.
      |
      | Si q = q0 + q1 i + q2 j + q3 k ,  alors
      |
      | phi = atan2( 2(q1q2+q0q3) , q0^2+q1^2 - q2^2-q3^2)
      | theta = asin(2q0q2-2q1q3)
      | psi = atan2( 2(q0q1+q2q3) , q0^2-q1^2 - q2^2+q3^2)
      mask Help: eval('OpenHelp(''A3_NG.mdl'', ''Help\html\A3_NG_Model_Quaternion2Euler.html'')');
  pqr2Quaternion : Subsystem  mask(pqr2Quaternion){Euler_Init=Euler_Init}
      mask prompts: Euler_Init "Angles d'Euler Initiaux"
      mask help:
      | Calcul du quaternion à partir des vitesses de rotation du missile et de
      | l'attidude initiale du missile.
      mask Help: eval('OpenHelp(''A3_NG.mdl'', ''Help\html\A3_NG_Model_pqr2Quaternion.html'')');
  Am : Outport  VectorParamsAs1DForOutWhenUnconnected=off
  Vm : Outport  Port=2  VectorParamsAs1DForOutWhenUnconnected=off
  Vi : Outport  Port=3  VectorParamsAs1DForOutWhenUnconnected=off
  Xi : Outport  Port=4  VectorParamsAs1DForOutWhenUnconnected=off
  pqr : Outport  Port=5  VectorParamsAs1DForOutWhenUnconnected=off
  Euler : Outport  Port=6  VectorParamsAs1DForOutWhenUnconnected=off
  wires:
  Ftot/1 -> Equations des forces/2(Faero)
  Equations des forces/1(Vb) -> Calcul de la vitesse engin dans le repère inertiel/1(Vb), Vm/1, [Vm]
  g/1 -> Pesanteur/2(g)
  Pesanteur/1(g_miss) -> Equations des forces/1(g)
  pqr2Quaternion/1(Quaternion) -> Calcul de la vitesse engin dans le repère inertiel/2(e0e1e2e3), Quaternion2Euler/1(Quaternion)
  Calcul de la vitesse engin dans le repère inertiel/1(Ve) -> Intégration de la vitesse dans le repère inertiel/1(Ve), Vi/1
  Quaternion2Euler/1(Euler) -> Pesanteur/1(Euler), Euler/1
  Intégration de la vitesse dans le repère inertiel/1(Xe) -> Xi/1
  Masse/1 -> Equations des forces/3(Masse)
  Equations des forces/2(Ab) -> Am/1, [Am]
  AlphaR/1 -> Calcul des pqr/3(AlphaR)
  BetaR/1 -> Calcul des pqr/4(BetaR)
  [Vm] -> Calcul des pqr/2(Vb)
  [Am] -> Calcul des pqr/1(Ab)
  Calcul des pqr/1(pqr) -> pqr/1, Equations des forces/4(pqr), pqr2Quaternion/1(pqr)
  pqr_force/1 -> Calcul des pqr/5(pqr_force)

== system MDR_AA_TMD_Intercepteur/Cible/Cible Cinématique v1.1/Pilote 2 axes Simulight à partir de gradient ==
  GcoV : Inport
  GcoH : Inport  Port=2
  Masse : Inport  Port=3
  Vm : Inport  Port=4
  Rho : Inport  Port=5
  Alpha commandé - Plan de tangage : Subsystem
  Beta commandé - Plan de lacet : Subsystem
  Masse1 : InportShadow  Port=3
  Norme : Subsystem  mask(Norme){}
      mask help: Calcul la norme quadratique d'un vecteur.
      mask Help: eval('OpenHelp(''A3_NG.mdl'', ''Help\html\A3_NG_Model_Norme.html'')');
  q\ : Subsystem
  Alphaco : Outport  VectorParamsAs1DForOutWhenUnconnected=off
  Betaco : Outport  Port=2  VectorParamsAs1DForOutWhenUnconnected=off
  wires:
  Vm/1 -> Norme/1(V)
  Norme/1(||V||) -> q\/1(||V||)
  Beta commandé - Plan de lacet/1(Betaco) -> Betaco/1
  Masse1/1 -> Beta commandé - Plan de lacet/2(Masse)
  GcoH/1 -> Beta commandé - Plan de lacet/1(GcoH)
  GcoV/1 -> Alpha commandé - Plan de tangage/1(GcoV)
  Alpha commandé - Plan de tangage/1(Alphaco) -> Alphaco/1
  Masse/1 -> Alpha commandé - Plan de tangage/2(Masse)
  q\/1(rsv2) -> [Pdyn]
  Rho/1 -> q\/2(Rho)
  [Pdyn] -> Alpha commandé - Plan de tangage/3(Pression_dynamique)
  [Pdyn] -> Beta commandé - Plan de lacet/3(Pression_dynamique)

== system MDR_AA_TMD_Intercepteur/Intercepteur_TMD/Auto-Directeur/Autodirecteur Parfait v1.0 ==
  Pos_Cible : Inport
  Vit_Cible : Inport  Port=2
  Pos_Miss : Inport  Port=3
  Vit_Miss : Inport  Port=4
  Euler : Inport  Port=5
  Calcul des angles site et gisement de la droite missile/but dans le repère missile : Subsystem
  Calcul des vitesses de défilements de la droite missile/but dans le repère missile : Subsystem
  Calcul du vecteur rotation instantané de la droite missile/but dans le repère inertiel : Subsystem
  "Changement de repère inertiel -> miss" : Subsystem
  Site et Gisement de la droite missile/but dans le repère inertiel : Subsystem
  Lambda_pt_y : Outport  VectorParamsAs1DForOutWhenUnconnected=off
  Lambda_pt_z : Outport  Port=2  VectorParamsAs1DForOutWhenUnconnected=off
  Psi_ad : Outport  Port=3  VectorParamsAs1DForOutWhenUnconnected=off
  Theta_ad : Outport  Port=4  VectorParamsAs1DForOutWhenUnconnected=off
  Lambda_ad : Outport  Port=5  VectorParamsAs1DForOutWhenUnconnected=off
  wires:
  Vit_Cible/1 -> Calcul du vecteur rotation instantané de la droite missile/but dans le repère inertiel/4(Vit_Cible_inert)
  Pos_Cible/1 -> Site et Gisement de la droite missile/but dans le repère inertiel/1(Pos_Cible_inert), Calcul du vecteur rotation instantané de la droite missile/but dans le repère inertiel/2(Pos_Cible_inert)
  Pos_Miss/1 -> Site et Gisement de la droite missile/but dans le repère inertiel/2(Pos_Miss_inert), Calcul du vecteur rotation instantané de la droite missile/but dans le repère inertiel/1(Pos_Miss_inert)
  Vit_Miss/1 -> Calcul du vecteur rotation instantané de la droite missile/but dans le repère inertiel/3(Vit_Miss_inert)
  Site et Gisement de la droite missile/but dans le repère inertiel/2(DMB) -> Calcul des angles site et gisement de la droite missile/but dans le repère missile/2(DMB)
  "Changement de repère inertiel -> miss"/2(Vmb_miss) -> Calcul des angles site et gisement de la droite missile/but dans le repère missile/1(Vmb_miss)
  Calcul du vecteur rotation instantané de la droite missile/but dans le repère inertiel/1(Omega_inert) -> "Changement de repère inertiel -> miss"/2(Omega_inert)
  "Changement de repère inertiel -> miss"/1(Omega_miss) -> Calcul des vitesses de défilements de la droite missile/but dans le repère missile/1(Omega_miss)
  Calcul des angles site et gisement de la droite missile/but dans le repère missile/1(Psi_ad) -> Psi_ad/1
  Calcul des vitesses de défilements de la droite missile/but dans le repère missile/1(wzad) -> Lambda_pt_z/1
  Calcul des vitesses de défilements de la droite missile/but dans le repère missile/2(wyad) -> Lambda_pt_y/1
  Site et Gisement de la droite missile/but dans le repère inertiel/1(Vmb_inert) -> "Changement de repère inertiel -> miss"/3(Vmb_inert)
  Euler/1 -> "Changement de repère inertiel -> miss"/1(Euler)
  Calcul des angles site et gisement de la droite missile/but dans le repère missile/2(Theta_ad) -> Theta_ad/1
  Calcul des angles site et gisement de la droite missile/but dans le repère missile/3(Lambda_ad) -> Lambda_ad/1

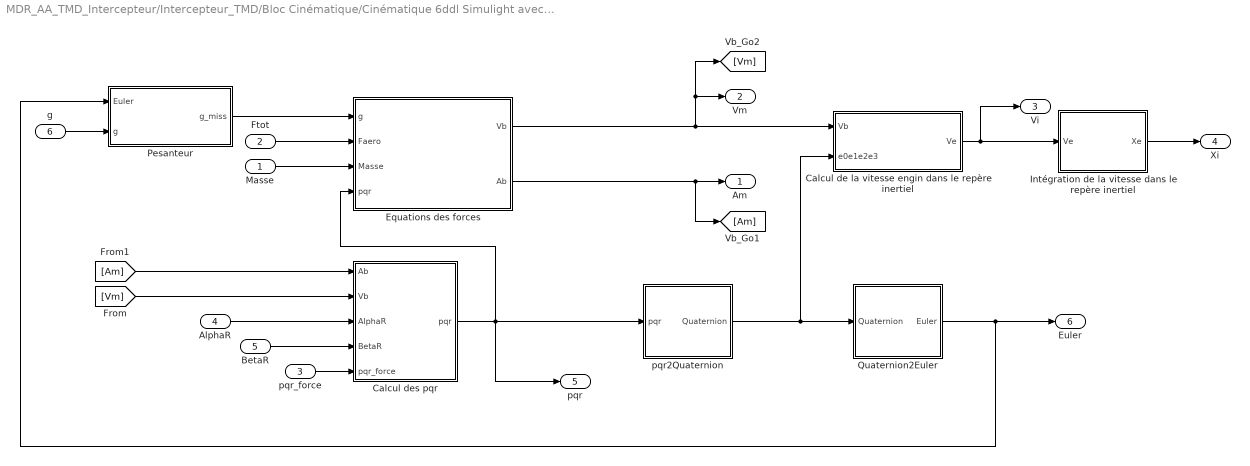
== system MDR_AA_TMD_Intercepteur/Intercepteur_TMD/Bloc Cinématique/Cinématique 6ddl Simulight avec pilotage en force ==
  Masse : Inport
  Ftot : Inport  Port=2
  pqr_force : Inport  Port=3
  AlphaR : Inport  Port=4
  BetaR : Inport  Port=5
  g : Inport  Port=6
  Calcul de la vitesse engin dans le repère inertiel : Subsystem
  Calcul des pqr : Subsystem
  Equations des forces : Subsystem
  Intégration de la vitesse dans le repère inertiel : Subsystem
  Pesanteur : Subsystem
  Quaternion2Euler : Subsystem  mask(Quaternion2Euler){}
      mask help:
      | Calcul des angles d'Euler (phi,theta,psi) à partir du quaternion q.
      |
      | Si q = q0 + q1 i + q2 j + q3 k ,  alors
      |
      | phi = atan2( 2(q1q2+q0q3) , q0^2+q1^2 - q2^2-q3^2)
      | theta = asin(2q0q2-2q1q3)
      | psi = atan2( 2(q0q1+q2q3) , q0^2-q1^2 - q2^2+q3^2)
      mask Help: eval('OpenHelp(''A3_NG.mdl'', ''Help\html\A3_NG_Model_Quaternion2Euler.html'')');
  pqr2Quaternion : Subsystem  mask(pqr2Quaternion){Euler_Init=Euler_Init}
      mask prompts: Euler_Init "Angles d'Euler Initiaux"
      mask help:
      | Calcul du quaternion à partir des vitesses de rotation du missile et de
      | l'attidude initiale du missile.
      mask Help: eval('OpenHelp(''A3_NG.mdl'', ''Help\html\A3_NG_Model_pqr2Quaternion.html'')');
  Am : Outport  VectorParamsAs1DForOutWhenUnconnected=off
  Vm : Outport  Port=2  VectorParamsAs1DForOutWhenUnconnected=off
  Vi : Outport  Port=3  VectorParamsAs1DForOutWhenUnconnected=off
  Xi : Outport  Port=4  VectorParamsAs1DForOutWhenUnconnected=off
  pqr : Outport  Port=5  VectorParamsAs1DForOutWhenUnconnected=off
  Euler : Outport  Port=6  VectorParamsAs1DForOutWhenUnconnected=off
  wires:
  Ftot/1 -> Equations des forces/2(Faero)
  Equations des forces/1(Vb) -> Calcul de la vitesse engin dans le repère inertiel/1(Vb), Vm/1, [Vm]
  g/1 -> Pesanteur/2(g)
  Pesanteur/1(g_miss) -> Equations des forces/1(g)
  pqr2Quaternion/1(Quaternion) -> Calcul de la vitesse engin dans le repère inertiel/2(e0e1e2e3), Quaternion2Euler/1(Quaternion)
  Calcul de la vitesse engin dans le repère inertiel/1(Ve) -> Intégration de la vitesse dans le repère inertiel/1(Ve), Vi/1
  Quaternion2Euler/1(Euler) -> Pesanteur/1(Euler), Euler/1
  Intégration de la vitesse dans le repère inertiel/1(Xe) -> Xi/1
  Masse/1 -> Equations des forces/3(Masse)
  Equations des forces/2(Ab) -> Am/1, [Am]
  AlphaR/1 -> Calcul des pqr/3(AlphaR)
  BetaR/1 -> Calcul des pqr/4(BetaR)
  [Vm] -> Calcul des pqr/2(Vb)
  [Am] -> Calcul des pqr/1(Ab)
  Calcul des pqr/1(pqr) -> pqr/1, Equations des forces/4(pqr), pqr2Quaternion/1(pqr)
  pqr_force/1 -> Calcul des pqr/5(pqr_force)

== system MDR_AA_TMD_Intercepteur/Intercepteur_TMD/Calculateur/Bloc Superviseur ==
  Bus_PM : Inport
  Bus_AD : Inport  Port=2
  Bus_DO : Inport  Port=3
  Bus_Senseurs : Inport  Port=4
  Bus Creator : BusCreator  Inputs=3
  Terminator1 : Terminator
  Terminator2 : Terminator
  Bus_Superviseur : Outport  VectorParamsAs1DForOutWhenUnconnected=off
  wires:
  Bus_PM/1 -> Terminator2/1
  Bus_Senseurs/1 -> Bus Creator/3  "Senseur"
  Bus_AD/1 -> Bus Creator/1
  Bus Creator/1 -> Bus_Superviseur/1
  Bus_DO/1 -> Terminator1/1
  [Global_Terre_Miss] -> Bus Creator/2

== system MDR_AA_TMD_Intercepteur/Intercepteur_TMD/Calculateur/Guidage ==
  Bus_Superviseur : Inport
  Bus Creator : BusCreator  Inputs=2
  Bus Selector : BusSelector  OutputSignals=Bus_AD.Lambda_pt_y,Bus_AD.Lambda_pt_z,Senseur.Vm,Bus_Terre.g
  Guidage en Naviguation Proportionnelle 2 axes : Subsystem  mask(Guidage en Navigation Proportionnelle 2 axes){N_V=3.8, N_H=3.8, Gmax=50}
      mask prompts: N_V "Gain de navigation proportionnelle (verticale)"; N_H "Gain de navigation proportionnelle (horrizontale)"; Gmax "Facteur de charge max (en g)"
      mask help: Loi de guidage en navigation propotionnelle deux axes avec compensation de la pesanteur.
      mask Help: eval('OpenHelp(''A3_NG.mdl'', ''Help\html\A3_NG_Model_Guidage_NP_2axes.html'')');
  Bus_Guidage : Outport  VectorParamsAs1DForOutWhenUnconnected=off
  wires:
  Bus_Superviseur/1 -> Bus Selector/1
  Bus Selector/2 -> Guidage en Naviguation Proportionnelle 2 axes/2(Lambda_pt_z)  "<Lambda_pt_z>"
  Bus Selector/1 -> Guidage en Naviguation Proportionnelle 2 axes/1(Lambda_pt_y)  "<Lambda_pt_y>"
  Bus Selector/3 -> Guidage en Naviguation Proportionnelle 2 axes/3(Vm)  "<Vm>"
  Bus Selector/4 -> Guidage en Naviguation Proportionnelle 2 axes/4(g)  "<g>"
  Guidage en Naviguation Proportionnelle 2 axes/2(GcoH) -> Bus Creator/2  "GcoH"
  Guidage en Naviguation Proportionnelle 2 axes/1(GcoV) -> Bus Creator/1  "GcoV"
  Bus Creator/1 -> Bus_Guidage/1  "Bus_Guidage"

== system MDR_AA_TMD_Intercepteur/Intercepteur_TMD/Calculateur/Pilotage ==
  Bus_Guidage : Inport
  Bus Creator : BusCreator  Inputs=2
  Bus Selector : BusSelector  OutputSignals=GcoV,GcoH
  Bus Selector1 : BusSelector  OutputSignals=Vson,Rho
  Bus Selector2 : BusSelector  OutputSignals=Masse
  Bus Selector3 : BusSelector  OutputSignals=Vm
  Pilote 2 axes Simulight avec prise en compte de la manoeuvrabilité max : Subsystem  mask(Pilote 2 axes Simulight){Lref=Aero_TMD.Lref, vMach=Aero_TMD.vMach, vAlpha=Aero_TMD.vAlpha, vBeta=Aero_TMD.vBeta, CN=Aero_TMD.CN, CY=Aero_TMD.CY, vMach_CNmax=Aero_TMD.vMach, CNmax=Aero_TMD.CNmax, vMach_CYmax=Aero_TMD.vMach, CYmax=Aero_TMD.CNmax}
      mask prompts: Lref "Longeur de référence (m)"; vMach "Plage des mach de l'étude"; vAlpha "Plage des incidences de l'étude"; vBeta "Plage des dérapages de l'étude"; CN "Table 2D des coefficients de portances CN"; CY "Table 2D des coefficients de portances CY"; vMach_CNmax "Plage de mach des coefficients équilibrés CNmax"; CNmax "Coefficients de portance max équilibré CNmax"; vMach_CYmax "Plage de mach des coefficients équilibrés CYmax"; CYmax "Coefficients de portance max équilibré CYmax"
      mask help: Calcul de l'incidence et du dérapage commandés permettant d'atteindre la consigne envoyée par le guidage.
      mask Help: eval('OpenHelp(''A3_NG.mdl'', ''Help\html\A3_NG_Model_Pilote_2axes_Simulight_Sature.html'')');
  Bus_Pilote : Outport  VectorParamsAs1DForOutWhenUnconnected=off
  wires:
  Bus Creator/1 -> Bus_Pilote/1  "Bus_Pilote"
  Pilote 2 axes Simulight avec prise en compte de la manoeuvrabilité max/1(Alphaco) -> Bus Creator/1  "AlphaC"
  Pilote 2 axes Simulight avec prise en compte de la manoeuvrabilité max/2(Betaco) -> Bus Creator/2  "BetaC"
  Bus_Guidage/1 -> Bus Selector/1
  Bus Selector/2 -> Pilote 2 axes Simulight avec prise en compte de la manoeuvrabilité max/2(GcoH)  "<GcoH>"
  Bus Selector/1 -> Pilote 2 axes Simulight avec prise en compte de la manoeuvrabilité max/1(GcoV)  "<GcoV>"
  [Global_Atm] -> Bus Selector1/1
  Bus Selector1/2 -> Pilote 2 axes Simulight avec prise en compte de la manoeuvrabilité max/6(Rho)  "<Rho>"
  Bus Selector1/1 -> Pilote 2 axes Simulight avec prise en compte de la manoeuvrabilité max/4(Vitesse_Son)  "<Vson>"
  [Global_Structure] -> Bus Selector2/1
  Bus Selector2/1 -> Pilote 2 axes Simulight avec prise en compte de la manoeuvrabilité max/3(Masse)  "<Masse>"
  Bus Selector3/1 -> Pilote 2 axes Simulight avec prise en compte de la manoeuvrabilité max/5(Vm)  "<Vm>"
  [Global_Cine_Missile] -> Bus Selector3/1

== system MDR_AA_TMD_Intercepteur/Intercepteur_TMD/Calculateur/Préparation de mission ==
  Ground : Ground
  Bus_PM : Outport  VectorParamsAs1DForOutWhenUnconnected=off
  wires:
  Ground/1 -> Bus_PM/1

== system MDR_AA_TMD_Intercepteur/Intercepteur_TMD/Forces-Moments/Aerodynamique 3D (CA//CY//CN) v1.0 ==
  Altitude : Inport
  Vm : Inport  Port=2
  Rho : Inport  Port=3
  Vson : Inport  Port=4
  AlphaR : Inport  Port=5
  BetaR : Inport  Port=6
  Ok_propu : Inport  Port=7
  Plan de lacet : Subsystem
  Plan de tangage : Subsystem
  Pression Dynamique Mach : Subsystem
  Trainée : Subsystem
  Vectorisation : Subsystem
  Faero : Outport  VectorParamsAs1DForOutWhenUnconnected=off
  wires:
  Trainée/1(A0) -> Vectorisation/1(Ax_Aero)
  Vectorisation/1(Faero) -> Faero/1
  Plan de lacet/1(Y0) -> Vectorisation/2(Ay_Aero)
  Plan de tangage/1(N0) -> Vectorisation/3(Az_Aero)
  Pression Dynamique Mach/1(rsv2) -> Plan de tangage/1(rsv2), Plan de lacet/1(rsv2), Trainée/1(rsv2)
  Pression Dynamique Mach/2(Mach) -> Plan de tangage/2(Mach), Plan de lacet/2(Mach), Trainée/2(Mach)
  Altitude/1 -> Trainée/4(Altitude)
  Ok_propu/1 -> Trainée/3(Ok_Propu)
  AlphaR/1 -> Plan de tangage/3(AlphaR)
  BetaR/1 -> Plan de lacet/3(BetaR)
  Vm/1 -> Pression Dynamique Mach/1(Vm)
  Rho/1 -> Pression Dynamique Mach/2(Rho)
  Vson/1 -> Pression Dynamique Mach/3(Vson)
